simulink model "Q2"  (R2020b)
settings: Solver=VariableStepAuto  StartTime=0.0  StopTime=60.0  RelTol=1e-3
libraries: simulink x1
settings Model: Creator=aloks  LastModifiedBy=aloks

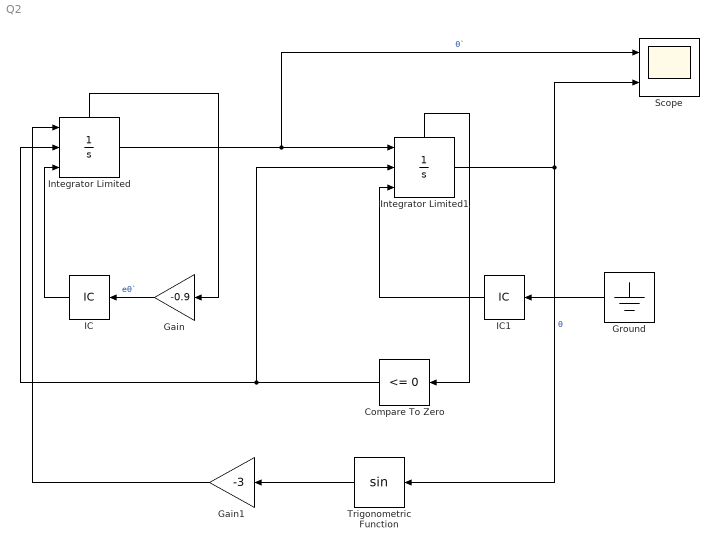
== system Q2 ==
  Compare To Zero : simulink/Logic and Bit Operations/Compare To Zero  relop=<=  OutDataTypeStr=boolean
  Gain : Gain  Gain=-0.9
  Gain1 : Gain  Gain=-3
  Ground : Ground
  IC : InitialCondition  Value=0
  IC1 : InitialCondition  Value=1.5707
  Integrator Limited : Integrator  ExternalReset=rising  InitialConditionSource=external  UpperSaturationLimit=100  LowerSaturationLimit=0  ShowStatePort=on
  Integrator Limited1 : Integrator  ExternalReset=rising  InitialConditionSource=external  LimitOutput=on  UpperSaturationLimit=100  LowerSaturationLimit=0  ShowStatePort=on
  Scope : Scope  NumInputPorts=2
  Trigonometric Function : Trigonometry
  wires:
  Integrator Limited/1 -> Scope/1, Integrator Limited1/1  "θ`"
  Integrator Limited1/1 -> Trigonometric Function/1, Scope/2  "θ"
  Integrator Limited/State -> Gain/1
  Gain/1 -> IC/1  "eθ`"
  IC/1 -> Integrator Limited/3
  Ground/1 -> IC1/1
  IC1/1 -> Integrator Limited1/3
  Integrator Limited1/State -> Compare To Zero/1
  Compare To Zero/1 -> Integrator Limited/2, Integrator Limited1/2
  Trigonometric Function/1 -> Gain1/1
  Gain1/1 -> Integrator Limited/1
